simulink model "System2"  (R2018b)
settings: Solver=VariableStepAuto  StartTime=0.0  StopTime=20  RelTol=1e-3
libraries: cstblocks x6, simulink x2
settings Model: Creator=Abraham Pérez  LastModifiedBy=Abraham Pérez

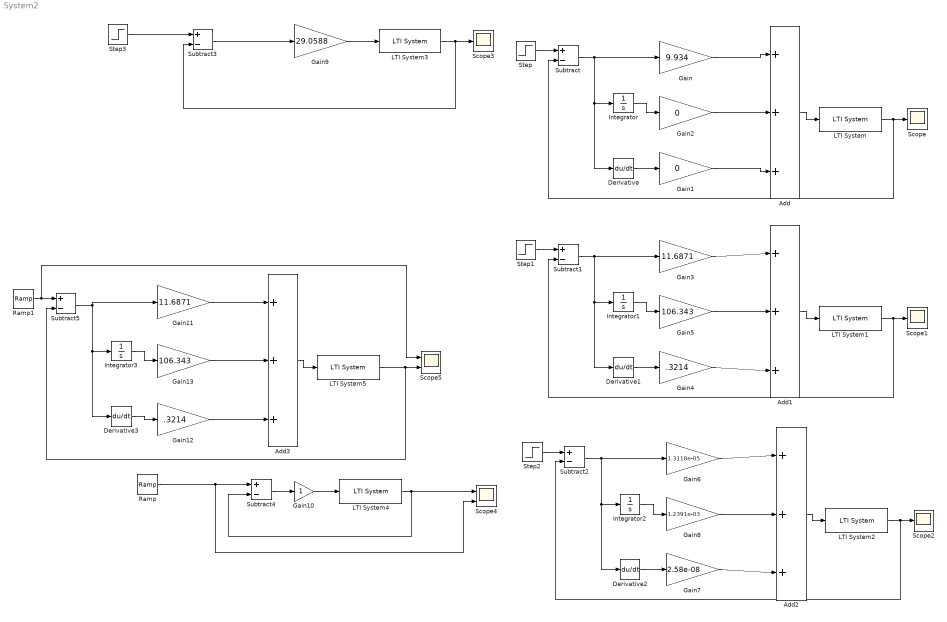
== system System2 ==
  Add{,1..3} (4 alike) : Sum  Inputs=+++
  Derivative{,1..3} (4 alike) : Derivative
  Gain : Gain  Gain=9.934
  Gain1 : Gain  Gain=0
  Gain10 : Gain
  Gain11 : Gain  Gain=11.6871
  Gain12 : Gain  Gain=.3214
  Gain13 : Gain  Gain=106.343
  Gain2 : Gain  Gain=0
  Gain3 : Gain  Gain=11.6871
  Gain4 : Gain  Gain=.3214
  Gain5 : Gain  Gain=106.343
  Gain6 : Gain  Gain=1.3118e-05
  Gain7 : Gain  Gain=2.58e-08
  Gain8 : Gain  Gain=1.2391e-03
  Gain9 : Gain  Gain=29.0588
  Integrator{,1..3} (4 alike) : Integrator
  LTI System{,1..5} (6 alike) : cstblocks/LTI System  sys=G2  IC=[]
  Ramp : simulink/Sources/Ramp  slope=1  start=5  InitialOutput=17
  Ramp1 : simulink/Sources/Ramp  slope=1  start=0  InitialOutput=17
  Scope{,1..3} (4 alike) : Scope
  Scope4 : Scope  NumInputPorts=2
  Scope5 : Scope  NumInputPorts=2
  Step : Step  Time=0  After=9  SampleTime=0
  Step1 : Step  Time=0  After=9  SampleTime=0
  Step2 : Step  Time=0  After=9  SampleTime=0
  Step3 : Step  Time=0  SampleTime=0
  Subtract{,1..5} (6 alike) : Sum  Inputs=+-
  wires:
  Add/1 -> LTI System/1
  LTI System/1 -> Subtract/2, Scope/1
  Gain1/1 -> Add/3
  Gain2/1 -> Add/2
  Gain/1 -> Add/1
  Integrator/1 -> Gain2/1
  Step/1 -> Subtract/1
  Subtract/1 -> Derivative/1, Integrator/1, Gain/1
  Derivative/1 -> Gain1/1
  Gain5/1 -> Add1/2
  LTI System1/1 -> Subtract1/2, Scope1/1
  Integrator1/1 -> Gain5/1
  Subtract1/1 -> Derivative1/1, Integrator1/1, Gain3/1
  Step1/1 -> Subtract1/1
  Gain4/1 -> Add1/3
  Derivative1/1 -> Gain4/1
  Gain3/1 -> Add1/1
  Add1/1 -> LTI System1/1
  Gain6/1 -> Add2/1
  Add2/1 -> LTI System2/1
  Gain7/1 -> Add2/3
  LTI System2/1 -> Subtract2/2, Scope2/1
  Integrator2/1 -> Gain8/1
  Gain8/1 -> Add2/2
  Derivative2/1 -> Gain7/1
  Step2/1 -> Subtract2/1
  Subtract2/1 -> Derivative2/1, Integrator2/1, Gain6/1
  Gain9/1 -> LTI System3/1
  Step3/1 -> Subtract3/1
  Subtract3/1 -> Gain9/1
  LTI System3/1 -> Subtract3/2, Scope3/1
  Ramp/1 -> Scope4/2, Subtract4/1
  Subtract4/1 -> Gain10/1
  LTI System4/1 -> Subtract4/2, Scope4/1
  Gain10/1 -> LTI System4/1
  Gain13/1 -> Add3/2
  Derivative3/1 -> Gain12/1
  Subtract5/1 -> Derivative3/1, Integrator3/1, Gain11/1
  LTI System5/1 -> Scope5/2, Subtract5/2
  Ramp1/1 -> Scope5/1, Subtract5/1
  Gain12/1 -> Add3/3
  Integrator3/1 -> Gain13/1
  Add3/1 -> LTI System5/1
  Gain11/1 -> Add3/1
